simulink model "FlapAct"  (R2024b)
settings: Solver=VariableStepAuto  StartTime=0.0  StopTime=10.0  RelTol=1e-3
settings Model: Creator=kkajak  LastModifiedBy=feder
settings SolverCC: AlgebraicLoopSolver=TrustRegion
settings DataIOCC: ReturnWorkspaceOutputs=off
settings DebuggingCC: UnconnectedInputMsg=warning  UnconnectedOutputMsg=warning  UnconnectedLineMsg=warning  ArithmeticOperatorsInVariantConditions=warning
settings ModelReferenceCC: EnableRefExpFcnMdlSchedulingChecks=on
settings SFSimCC: SimUseLocalCustomCode=off  CustomCodeUndefinedFunction=UseInterfaceOnly
settings RTWCC: RTWUseLocalCustomCode=off  GPUComputeCapability=3.5
settings CodeAppCC: StateflowObjectComments=on

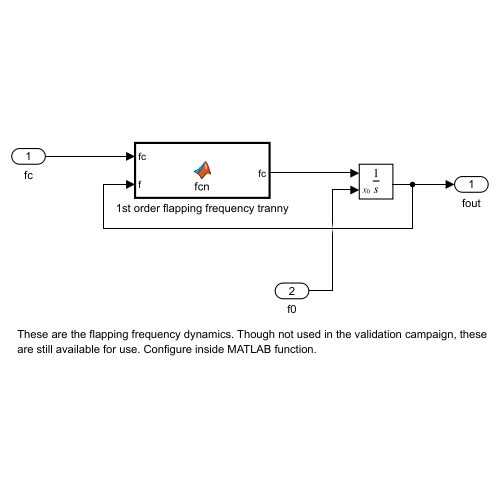
[thumbnail: Simulink's stored preview of the top-level diagram]
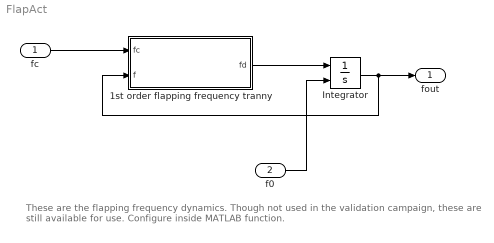
== system FlapAct ==
  note: These are the flapping frequency dynamics. Though not used in the validation campaign, these
      | are still available for use. Configure inside MATLAB function.
  fc : Inport
  f0 : Inport  Port=2
  1st order flapping frequency tranny : MATLAB Function  TreatAsAtomicUnit=on
  Integrator : Integrator  InitialConditionSource=external
  fout : Outport
  wires:
  1st order flapping frequency tranny/1(fd) -> Integrator/1
  f0/1 -> Integrator/2
  Integrator/1 -> fout/1, 1st order flapping frequency tranny/2(f)
  fc/1 -> 1st order flapping frequency tranny/1(fc)

== matlab function FlapAct/1st order flapping frequency tranny ==
  data: fc input; fd output; f input
function fd = fcn(fc,f)

%fd = 11.04*fc - 12.56*f;
fd = 12.56*fc - 12.56*f;
